simulink model "bus_collision"  (Simulink 8.0)
settings: Solver=ode45  StartTime=0.0  StopTime=10.0  RelTol=1e-3
settings Model: Creator=transima  LastModifiedBy=transima

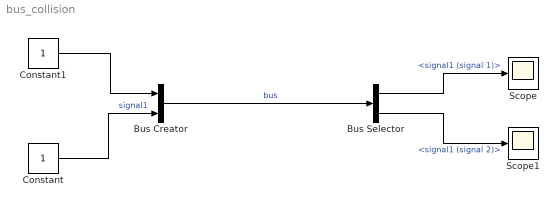
== system bus_collision ==
  Bus Creator : BusCreator  Inputs=2
  Bus Selector : BusSelector  OutputSignals=signal1 (signal 1),signal1 (signal 2)
  Constant : Constant
  Constant1 : Constant
  Scope : Scope
  Scope1 : Scope
  wires:
  Constant1/1 -> Bus Creator/1
  Bus Creator/1 -> Bus Selector/1  "bus"
  Bus Selector/1 -> Scope/1  "<signal1 (signal 1)>"
  Bus Selector/2 -> Scope1/1  "<signal1 (signal 2)>"
  Constant/1 -> Bus Creator/2  "signal1"
